simulink model "w2project4"  (R2020b)
settings: Solver=VariableStepAuto  StartTime=0.0  StopTime=10.0  RelTol=1e-3
settings Model: DataDictionary=w2project4.sldd  Creator=rutvi  LastModifiedBy=rutvi

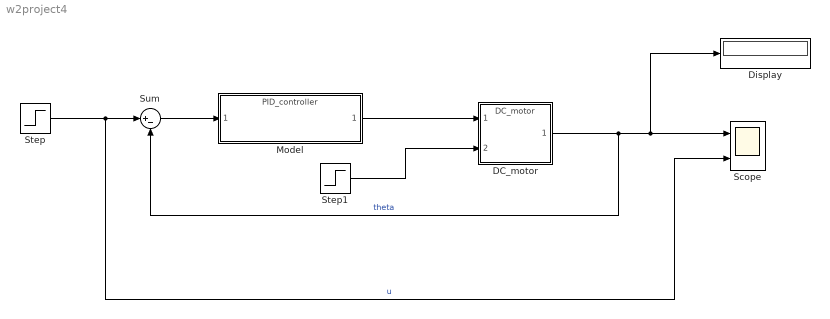
== system w2project4 ==
  DC_motor : ModelReference  ModelNameDialog=DC_motor  SimulationMode=Normal  ModelReferenceVersion=1.5
  Display : Display
  Model : ModelReference  ModelNameDialog=PID_controller.slx  SimulationMode=Normal  ModelReferenceVersion=1.7
  Scope : Scope  NumInputPorts=2
  Step : Step  SampleTime=0
  Step1 : Step  After=-0.01  SampleTime=0
  Sum : Sum  Inputs=|+-
  wires:
  Step/1 -> Scope/2, Sum/1  "u"
  DC_motor/1 -> Display/1, Scope/1, Sum/2  "theta"
  Step1/1 -> DC_motor/2
  Model/1 -> DC_motor/1
  Sum/1 -> Model/1
